simulink model "test"  (R2015a)
settings: Solver=ode15s  StartTime=0.0  StopTime=40  RelTol=1e-6  AbsTol=1e-9
InitFcn:
  | delta = 20;
  | kmu = 50;
  | 
  | beta = 0;
  | %beta = -10;
  | gamma = 0;
  | gamma = 5;
settings Model: Creator=ironi  LastModifiedBy=ironi
settings HardwareCC: ProdBitPerLong=64  ProdBitPerPointer=64  ProdWordSize=64  ProdHWDeviceType=Generic->64-bit Embedded Processor (LP64)

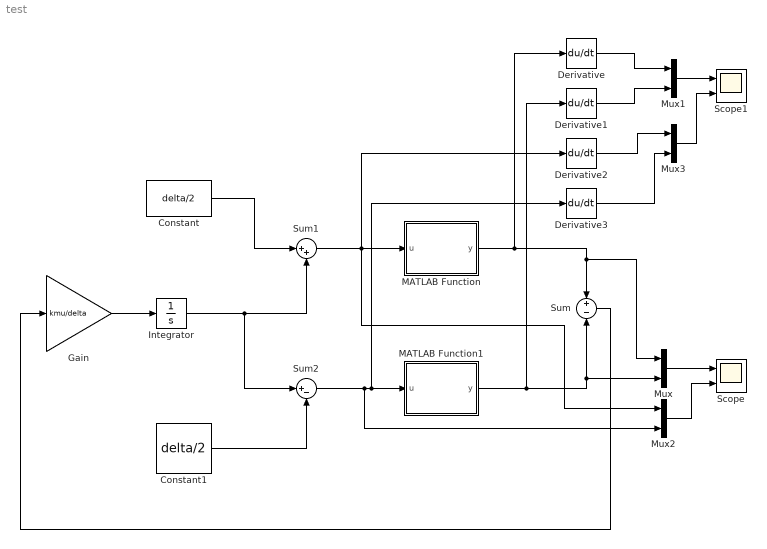
== system test ==
  Constant : Constant  Value=delta/2
  Constant1 : Constant  Value=delta/2
  Derivative{,1..3} (4 alike) : Derivative
  Gain : Gain  Gain=kmu/delta
  Integrator : Integrator  InitialCondition=30
  MATLAB Function : MATLAB Function  TreatAsAtomicUnit=on
  MATLAB Function1 : MATLAB Function  TreatAsAtomicUnit=on
  Mux{,1..3} (4 alike) : Mux  Inputs=2
  Scope : Scope  NumInputPorts=2
      settings: YMin=-5~-5  YMax=5~5
  Scope1 : Scope  NumInputPorts=2
      settings: YMin=-5~-5  YMax=5~5
  Sum : Sum  Inputs=+|-
  Sum1 : Sum  Inputs=|++
  Sum2 : Sum  Inputs=|+-
  wires:
  MATLAB Function/1(y) -> Derivative/1, Mux/1, Sum/1
  MATLAB Function1/1(y) -> Derivative1/1, Mux/2, Sum/2
  Sum/1 -> Gain/1
  Gain/1 -> Integrator/1
  Sum1/1 -> Derivative2/1, Mux2/1, MATLAB Function/1(u)
  Constant/1 -> Sum1/1
  Integrator/1 -> Sum2/1, Sum1/2
  Mux/1 -> Scope/1
  Constant1/1 -> Sum2/2
  Sum2/1 -> Mux2/2, Derivative3/1, MATLAB Function1/1(u)
  Mux1/1 -> Scope1/1
  Derivative/1 -> Mux1/1
  Derivative1/1 -> Mux1/2
  Mux2/1 -> Scope/2
  Mux3/1 -> Scope1/2
  Derivative2/1 -> Mux3/1
  Derivative3/1 -> Mux3/2

== matlab function test/MATLAB Function1 ==
  data: u input; y output; beta parameter; gamma parameter
function y = fcn(u, beta, gamma)
%#codegen

% beta = 0;
% % beta = -10;
% gamma = 0;
% gamma = 5;

Dopt = zeros(1,2);
Jopt = zeros(1,2);

Dopt(1) = 100;
Jopt(1) = 20;
Dopt(2) = 100 - beta;
Jopt(2) = 20  + gamma;

y = -0.002 * (u - Dopt(2))^2 + Jopt(2);

== matlab function test/MATLAB Function ==
  data: u input; y output; beta parameter; gamma parameter
function y = fcn(u, beta, gamma)
%#codegen

% beta = 0;
% % beta = -10;
% gamma = 0;
% gamma = 5;

Dopt = zeros(1,2);
Jopt = zeros(1,2);

Dopt(1) = 100;
Jopt(1) = 20;
Dopt(2) = 100 - beta;
Jopt(2) = 20  + gamma;

y = -0.002 * (u - Dopt(1))^2 + Jopt(1);
